simulink model "UKF_MDL"  (R2013a)
settings: Solver=VariableStepDiscrete  StartTime=0.0  StopTime=50  RelTol=1e-3
settings Model: Creator=Aleksandr  LastModifiedBy=Aleksandr

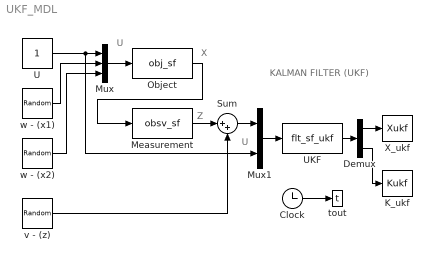
== system UKF_MDL ==
  note: KALMAN FILTER
      | (UKF)
  note: U
  note: Z
  note: U
  note: X
  Clock : Clock
      settings: Decimation=100
  Demux : Demux  Outputs=2
  K_ukf : ToWorkspace  VariableName=Kukf  SampleTime=-1
  Measurement : S-Function  FunctionName=obsv_sf  EnableBusSupport=off
  Mux : Mux  Inputs=3
  Mux1 : Mux  Inputs=2
  Object : S-Function  FunctionName=obj_sf  EnableBusSupport=off
  Sum : Sum  Inputs=|++
  U : Constant
  UKF : S-Function  FunctionName=flt_sf_ukf  EnableBusSupport=off
  X_ukf : ToWorkspace  VariableName=Xukf  SampleTime=-1
  tout : ToWorkspace  VariableName=t  SampleTime=-1
  v - (z) : RandomNumber  Variance=1.15  SampleTime=0.1
  w - (x1) : RandomNumber  Variance=0.01  SampleTime=0.1
  w - (x2) : RandomNumber  Variance=0.04  SampleTime=0.1
  wires:
  Mux/1 -> Object/1
  w - (x2)/1 -> Mux/3
  w - (x1)/1 -> Mux/2
  Measurement/1 -> Sum/1
  v - (z)/1 -> Sum/2
  Mux1/1 -> UKF/1
  Sum/1 -> Mux1/1
  U/1 -> Mux1/2, Mux/1
  Clock/1 -> tout/1
  Object/1 -> Measurement/1
  Demux/1 -> X_ukf/1
  Demux/2 -> K_ukf/1
  UKF/1 -> Demux/1
